simulink model "Junctions"  (Simulink 7.4)
settings: Solver=ode45  StartTime=0.0  StopTime=10.0  RelTol=1e-3
settings Model: Creator=dread  LastModifiedBy=dread

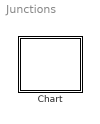
== system Junctions ==
  Chart : Stateflow chart

== stateflow chart Chart ==
  state Start
  state End
  Start -> (junction 5)
  (junction 5) -> (junction 6) [order 1]
  (junction 6) -> End
  (junction 5) -> (junction 6) [order 2]
